simulink model "Project5"  (R2024b)
settings: Solver=VariableStepAuto  StartTime=0.0  StopTime=Sim_Time  RelTol=1e-3
values from neighbouring files (symbols this model uses):
  Cn = 2.3 * 3600    (= 8280)    [Project5_run.m]
  I = 2.3    [Project5_run.m]
  OCV = Data(:,2)    [Project5_run.m]
  R_Charge = Data(:,3)    [Project5_run.m]
  R_Discharge = Data(:,4)    [Project5_run.m]
  SOC = Data(:,1)    [Project5_run.m]
settings Model: Creator=szala  LastModifiedBy=szala

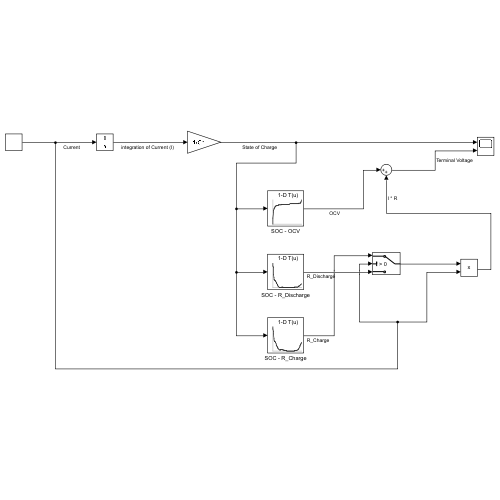
[thumbnail: Simulink's stored preview of the top-level diagram]
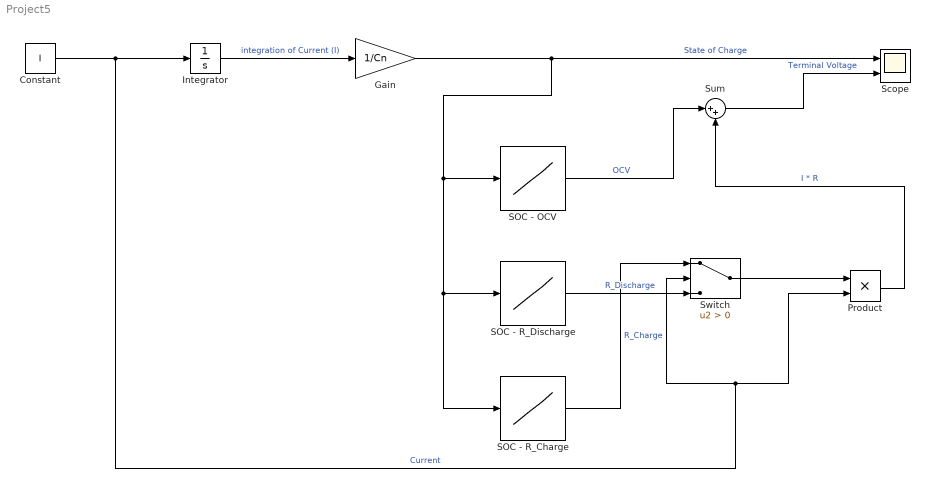
== system Project5 ==
  Constant : Constant  Value=I
  Gain : Gain  Gain=1/Cn
  Integrator : Integrator
  Product : Product
  SOC - OCV : Lookup_n-D  NumberOfTableDimensions=1  BreakpointsForDimension1=SOC  Table=OCV  InternalRulePriority=Speed  RndMeth=Simplest
  SOC - R_Charge : Lookup_n-D  NumberOfTableDimensions=1  BreakpointsForDimension1=SOC  Table=R_Charge  InternalRulePriority=Speed  RndMeth=Simplest
  SOC - R_Discharge : Lookup_n-D  NumberOfTableDimensions=1  BreakpointsForDimension1=SOC  Table=R_Discharge  InternalRulePriority=Speed  RndMeth=Simplest
  Scope : Scope  NumInputPorts=2
  Sum : Sum  Inputs=|++
  Switch : Switch  Criteria=u2 > Threshold  SaturateOnIntegerOverflow=off  InputSameDT=off
  wires:
  Constant/1 -> Product/2, Switch/2, Integrator/1  "Current"
  Integrator/1 -> Gain/1  "integration of Current (I)"
  Gain/1 -> SOC - R_Charge/1, SOC - R_Discharge/1, SOC - OCV/1, Scope/1  "State of Charge"
  SOC - OCV/1 -> Sum/1  "OCV"
  Product/1 -> Sum/2  "I * R"
  Sum/1 -> Scope/2  "Terminal Voltage"
  Switch/1 -> Product/1
  SOC - R_Discharge/1 -> Switch/3  "R_Discharge"
  SOC - R_Charge/1 -> Switch/1  "R_Charge"
